simulink model "Model_5_2"  (R2015b)
settings: Solver=VariableStepAuto  StartTime=0.0  StopTime=10.0  RelTol=1e-3
libraries: simulink x2
settings Model: Creator=etsu  LastModifiedBy=etsu

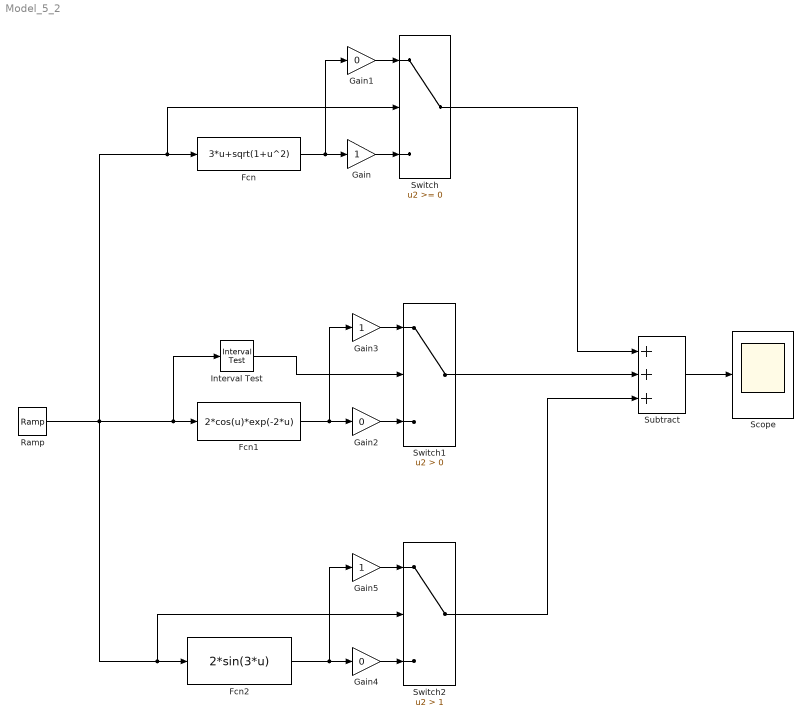
== system Model_5_2 ==
  Fcn : Fcn  Expr=3*u+sqrt(1+u^2)
  Fcn1 : Fcn  Expr=2*cos(u)*exp(-2*u)
  Fcn2 : Fcn  Expr=2*sin(3*u)
  Gain : Gain
  Gain1 : Gain  Gain=0
  Gain2 : Gain  Gain=0
  Gain3 : Gain
  Gain4 : Gain  Gain=0
  Gain5 : Gain
  Interval Test : simulink/Logic and Bit Operations/Interval Test  IntervalClosedRight=on  uplimit=1  IntervalClosedLeft=on  lowlimit=0  OutDataTypeStr=boolean
  Ramp : simulink/Sources/Ramp  slope=1  start=0  X0=-5
  Scope : Scope
  Subtract : Sum  Inputs=+++
  Switch : Switch
  Switch1 : Switch  Criteria=u2 > Threshold
  Switch2 : Switch  Criteria=u2 > Threshold  Threshold=1
  wires:
  Fcn/1 -> Gain1/1, Gain/1
  Gain1/1 -> Switch/1
  Gain/1 -> Switch/3
  Ramp/1 -> Fcn/1, Switch/2, Switch2/2, Fcn2/1, Interval Test/1, Fcn1/1
  Subtract/1 -> Scope/1
  Switch/1 -> Subtract/1
  Fcn1/1 -> Gain3/1, Gain2/1
  Gain3/1 -> Switch1/1
  Gain2/1 -> Switch1/3
  Interval Test/1 -> Switch1/2
  Switch1/1 -> Subtract/2
  Fcn2/1 -> Gain5/1, Gain4/1
  Gain5/1 -> Switch2/1
  Gain4/1 -> Switch2/3
  Switch2/1 -> Subtract/3
